simulink model "AFE"  (Simulink 8.7)
settings: Solver=ode23t  StartTime=0  StopTime=.2  MaxStep=.1e-6  RelTol=1e-4  AbsTol=1e-5
InitFcn:
  | clear all
  | VSI_AFE_parameters_G1_s
values from neighbouring files (symbols this model uses):
  Cdc_afe = 105e-6    (= 0.000105)    [VSI_AFE_parameters_G1_s.m]
  DeadTime = 0.5e-6    (= 5e-07)    [VSI_AFE_parameters_G1_s.m]
  f = 400    [VSI_AFE_parameters_G1_s.m]
  Lboost_a = 500e-6    (= 0.0005)    [VSI_AFE_parameters_G1_s.m]
  Lboost_b = 490e-6    (= 0.00049)    [VSI_AFE_parameters_G1_s.m]
  Lboost_c = 510e-6    (= 0.00051)    [VSI_AFE_parameters_G1_s.m]
  LCdc_afe = 0.65e-6    (= 6.5e-07)    [VSI_AFE_parameters_G1_s.m]
  PWM_Cycle = 4000    [VSI_AFE_parameters_G1_s.m]
  RCdc_afe = 0.049    [VSI_AFE_parameters_G1_s.m]
  Rdc = 96    [VSI_AFE_parameters_G1_s.m]
  RLboost_a = 0.080    (= 0.08)    [VSI_AFE_parameters_G1_s.m]
  RLboost_b = 0.084    [VSI_AFE_parameters_G1_s.m]
  RLboost_c = 0.110    (= 0.11)    [VSI_AFE_parameters_G1_s.m]
  Tsw = 1/fsw    (= 5e-05)    [VSI_AFE_parameters_G1_s.m]
  Vfd = 0.75    [VSI_AFE_parameters_G1_s.m]
  Vfs = 1.0    (= 1)    [VSI_AFE_parameters_G1_s.m]
  Vsm = Vse*sqrt(2)    [VSI_AFE_parameters_G1_s.m]
undefined symbols (not defined in the file or in its folder): Cdc, Ldc
libraries: powerlib x28, cstblocks x10, simulink x2
settings Model: Creator=marko  LastModifiedBy=mchssbw3
settings SolverCC: MaxConsecutiveMinStep=10  ZeroCrossAlgorithm=Adaptive  AlgebraicLoopSolver=LineSearch
settings DataIOCC: LimitDataPoints=off  SaveFinalState=on  SignalLoggingSaveFormat=ModelDataLogs
settings OptimizationCC: ExpressionDepthLimit=2147483647
settings DebuggingCC: IgnoredZcDiagnostic=none  SolverPrmCheckMsg=warning  FcnCallInpInsideContextMsg=UseLocalSettings  StateNameClashWarn=warning  StrictBusMsg=Warning
settings GRTTargetCC: CombineOutputUpdateFcns=off  GRTInterface=on

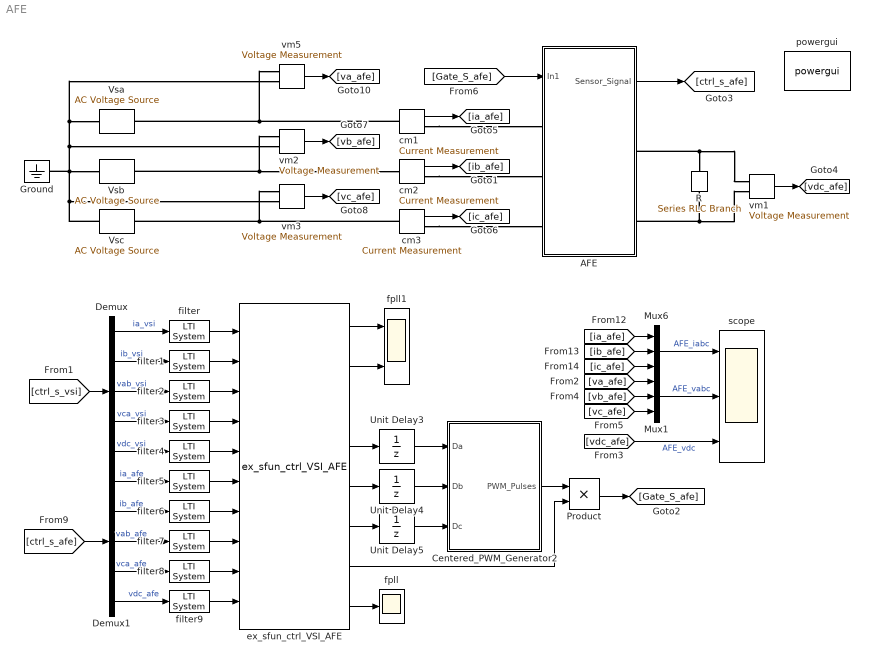
== system AFE ==
  AFE : Subsystem
  Centered_PWM_Generator2 : Subsystem
  Demux : Demux  Outputs=5
  Demux1 : Demux  Outputs=5
  Ground : powerlib/Elements/Ground  LConnTagsString=a
  Mux1 : Mux  Inputs=3
  Mux6 : Mux  Inputs=3
  Product : Product  RndMeth=Zero
  R : powerlib/Elements/Series RLC Branch  LConnTagsString=__new0  RConnTagsString=__new0  BranchType=R  Resistance=Rdc  Inductance=Ldc  SetiL0=off  InitialCurrent=0  Capacitance=Cdc  Setx0=off  InitialVoltage=0  Measurements=None
  Unit Delay3 : UnitDelay  SampleTime=-1
  Unit Delay4 : UnitDelay  SampleTime=-1
  Unit Delay5 : UnitDelay  SampleTime=Tsw
  Vsa : powerlib/Electrical Sources/AC Voltage Source  Amplitude=Vsm  Phase=0  Frequency=f  SampleTime=0  Measurements=None  BusType=swing  Pref=10e3  Qref=0  Qmin=-inf  Qmax=+inf
  Vsb : powerlib/Electrical Sources/AC Voltage Source  Amplitude=Vsm  Phase=0-120  Frequency=f  SampleTime=0  Measurements=None  BusType=swing  Pref=10e3  Qref=0  Qmin=-inf  Qmax=+inf
  Vsc : powerlib/Electrical Sources/AC Voltage Source  Amplitude=Vsm  Phase=0+120  Frequency=f  SampleTime=0  Measurements=None  BusType=swing  Pref=10e3  Qref=0  Qmin=-inf  Qmax=+inf
  cm1 : powerlib/Measurements/Current Measurement  PhasorSimulation=off  OutputType=Complex  PSBequivalent=0
  cm2 : powerlib/Measurements/Current Measurement  PhasorSimulation=off  OutputType=Complex  PSBequivalent=0
  cm3 : powerlib/Measurements/Current Measurement  PhasorSimulation=off  OutputType=Complex  PSBequivalent=0
  ex_sfun_ctrl_VSI_AFE : S-Function  FunctionName=ex_sfun_ctrl_VSI_AFE  SFunctionDeploymentMode=off  EnableBusSupport=off  mask(Legacy Function){SFunctionSpec=void epwm1_isr(double y1[1], double y2[1], double y3[1], double y4[1], double y5[1], double y6[1], double y7[1], double y8[1], double y9[1], double u1, double u2, double u3, double u4, double u5, double u6, double u7, double u8, double u9, double u10), ShowSpec=off}
      mask prompts: ShowSpec "Display function specification"
      mask help:
      | This block allows you to call the legacy functions specified by the following Legacy Code Tool definition:
      | def.SFunctionName = 'ex_sfun_ctrl_VSI_AFE';
      | def.OutputFcnSpec = 'void epwm1_isr(double y1[1], double y2[1], double y3[1], double y4[1], double y5[1], double y6[1], double y7[1], double y8[1], double y9[1], double u1, double u2, double u3, double u4, double u5, double u6, double u7, double u8, double u9, double u10)';
      | def.HeaderFiles = {'math.h'};
      | def.SourceFiles = {'epwm1_isr.c'};
      | def.SampleTime = 5e-005;
      mask Help: <p>This block was generated automatically by the Legacy Code Tool. For detailed help on this tool, call<a href="matlab:legacy_code('help')"> legacy_code('help')</a>.</p>
      mask Callback ShowSpec:
      | if strcmp(get_param(gcbh, 'ShowSpec'), 'on')
      |   set_param(gcbh, 'MaskDisplay', sprintf('fprintf(''%s'');', get_param(gcbh, 'SFunctionSpec')));
      | else
      |   set_param(gcbh, 'MaskDisplay', sprintf('fprintf(''%s'');', get_param(gcbh, 'FunctionName')));
      | end
      mask Display: fprintf('ex_sfun_ctrl_VSI_AFE');
  filter{,1..9} (10 alike) : cstblocks/LTI System  sys=tf_filter  IC=[]
  fpll : Scope
  fpll1 : Scope  NumInputPorts=2
  powergui : powerlib/powergui  Priority=1  SimulationMode=Continuous  SolverType=Tustin  SampleTime=100e-9  frequency=60  SPID=on  DisableSnubberDevices=off  DisableRonSwitches=off  DisableVfSwitches=off  SwTol=0  DisplayEquations=off  Interpol=off  ExternalGateDelay=off  methode=off  Ts=0  FunctionMessages=off  echomessages=off  HookPort=off  EnableUseOfTLC=off  x0status=blocks  frequencyindice=0  Pbase=100e6  ErrMax=1e-4  Iterations=50  UnitsV=kV  UnitsW=MW  buscounter=0  RestoreLinks=warning  ResistiveCurrentMeasurement=off  Frange=[0:2:500]  Ylog=off  Xlog=on  ShowGrid=off  save=off  variable=ZData  structure=iabc  ZoomFFT=off  StartTime=0.1  cycles=2  DisplayStyle=2  fundamental=400  FreqAxis=off  MaxFrequency=100000  frequencyindicesteady=400  RmsSteady=1  display=off
  scope : Scope  NumInputPorts=3
  vm{1..3,5} (4 alike) : powerlib/Measurements/Voltage Measurement  PhasorSimulation=off  OutputType=Complex  PSBequivalent=0
  wires:
  vm5/1 -> [va_afe]
  [ia_afe] -> Mux6/1
  [ib_afe] -> Mux6/2
  [ic_afe] -> Mux6/3
  Mux6/1 -> scope/1  "AFE_iabc"
  Demux/1 -> filter/1  "ia_vsi"
  Demux/2 -> filter1/1  "ib_vsi"
  Demux/3 -> filter2/1  "vab_vsi"
  Demux/4 -> filter3/1  "vca_vsi"
  Demux/5 -> filter4/1  "vdc_vsi"
  [ctrl_s_vsi] -> Demux/1
  Demux1/1 -> filter5/1  "ia_afe"
  Demux1/2 -> filter6/1  "ib_afe"
  Demux1/3 -> filter7/1  "vab_afe"
  Demux1/4 -> filter8/1  "vca_afe"
  Demux1/5 -> filter9/1  "vdc_afe"
  [ctrl_s_afe] -> Demux1/1
  [Gate_S_afe] -> AFE/1(In1)
  AFE/1(Sensor_Signal) -> [ctrl_s_afe]
  Unit Delay3/1 -> Centered_PWM_Generator2/1(Da)
  Unit Delay4/1 -> Centered_PWM_Generator2/2(Db)
  Unit Delay5/1 -> Centered_PWM_Generator2/3(Dc)
  ex_sfun_ctrl_VSI_AFE/4 -> Unit Delay3/1
  ex_sfun_ctrl_VSI_AFE/5 -> Unit Delay4/1
  ex_sfun_ctrl_VSI_AFE/6 -> Unit Delay5/1
  filter/1 -> ex_sfun_ctrl_VSI_AFE/1
  filter1/1 -> ex_sfun_ctrl_VSI_AFE/2
  filter2/1 -> ex_sfun_ctrl_VSI_AFE/3
  filter3/1 -> ex_sfun_ctrl_VSI_AFE/4
  filter4/1 -> ex_sfun_ctrl_VSI_AFE/5
  filter5/1 -> ex_sfun_ctrl_VSI_AFE/6
  filter6/1 -> ex_sfun_ctrl_VSI_AFE/7
  filter7/1 -> ex_sfun_ctrl_VSI_AFE/8
  filter8/1 -> ex_sfun_ctrl_VSI_AFE/9
  filter9/1 -> ex_sfun_ctrl_VSI_AFE/10
  Centered_PWM_Generator2/1(PWM_Pulses) -> Product/1
  Product/1 -> [Gate_S_afe]
  ex_sfun_ctrl_VSI_AFE/7 -> Product/2
  ex_sfun_ctrl_VSI_AFE/8 -> fpll/1
  vm1/1 -> [vdc_afe]
  cm1/1 -> [ia_afe]
  Mux1/1 -> scope/2  "AFE_vabc"
  [vdc_afe] -> scope/3  "AFE_vdc"
  cm2/1 -> [ib_afe]
  cm3/1 -> [ic_afe]
  vm2/1 -> [vb_afe]
  vm3/1 -> [vc_afe]
  [va_afe] -> Mux1/1
  [vb_afe] -> Mux1/2
  [vc_afe] -> Mux1/3
  ex_sfun_ctrl_VSI_AFE/1 -> fpll1/1
  ex_sfun_ctrl_VSI_AFE/2 -> fpll1/2
  connections:
  AFE/RConn2 -- R/RConn1 -- vm1/LConn2
  AFE/RConn1 -- R/LConn1 -- vm1/LConn1
  cm1/RConn1 -- AFE/LConn1
  cm2/RConn1 -- AFE/LConn2
  cm3/RConn1 -- AFE/LConn3
  Vsb/LConn1 -- Ground/LConn1 -- Vsc/LConn1 -- vm3/LConn2 -- Vsa/LConn1 -- vm5/LConn2 -- vm2/LConn2
  Vsa/RConn1 -- cm1/LConn1 -- vm5/LConn1
  Vsb/RConn1 -- vm2/LConn1 -- cm2/LConn1
  Vsc/RConn1 -- cm3/LConn1 -- vm3/LConn1

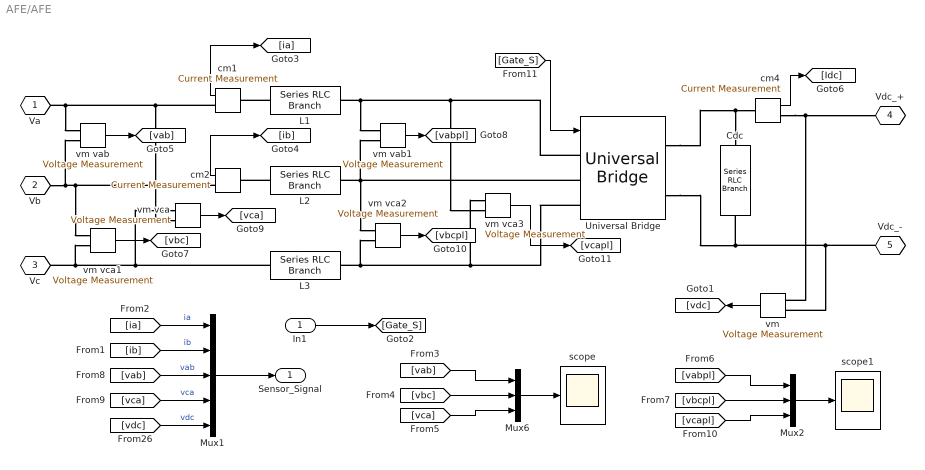
== system AFE/AFE ==
  In1 : Inport
  Cdc : powerlib/Elements/Series RLC Branch  LConnTagsString=__new0  RConnTagsString=__new0  BranchType=RC  Resistance=RCdc_afe  Inductance=LCdc_afe  SetiL0=off  InitialCurrent=0  Capacitance=Cdc_afe  Setx0=off  InitialVoltage=0  Measurements=None
  L1 : powerlib/Elements/Series RLC Branch  LConnTagsString=__new0  RConnTagsString=__new0  BranchType=RL  Resistance=RLboost_a  Inductance=Lboost_a  SetiL0=off  InitialCurrent=0  Capacitance=1e-6  Setx0=off  InitialVoltage=0  Measurements=None
  L2 : powerlib/Elements/Series RLC Branch  LConnTagsString=__new0  RConnTagsString=__new0  BranchType=RL  Resistance=RLboost_b  Inductance=Lboost_b  SetiL0=off  InitialCurrent=0  Capacitance=1e-6  Setx0=off  InitialVoltage=0  Measurements=None
  L3 : powerlib/Elements/Series RLC Branch  LConnTagsString=__new0  RConnTagsString=__new0  BranchType=RL  Resistance=RLboost_c  Inductance=Lboost_c  SetiL0=off  InitialCurrent=0  Capacitance=1e-6  Setx0=off  InitialVoltage=0  Measurements=None
  Mux1 : Mux  Inputs=5
  Mux2 : Mux  Inputs=3
  Mux6 : Mux  Inputs=3
  Universal Bridge : powerlib/Power Electronics/Universal Bridge  Arms=3  SnubberResistance=inf  SnubberCapacitance=inf  Device=IGBT / Diodes  Ron=Rsd  Lon=0  ForwardVoltages=[Vfs Vfd]  ForwardVoltage=0  GTOparameters=[ 10e-6 , 20e-6 ]  IGBTparameters=[ 0, 0 ]  Measurements=None  Measurements_2=None  converterType=Rectifier
  cm1 : powerlib/Measurements/Current Measurement  PhasorSimulation=off  OutputType=Complex  PSBequivalent=0
  cm2 : powerlib/Measurements/Current Measurement  PhasorSimulation=off  OutputType=Complex  PSBequivalent=0
  cm4 : powerlib/Measurements/Current Measurement  PhasorSimulation=off  OutputType=Complex  PSBequivalent=0
  scope : Scope
  scope1 : Scope
  vm : powerlib/Measurements/Voltage Measurement  PhasorSimulation=off  OutputType=Complex  PSBequivalent=0
  vm vab : powerlib/Measurements/Voltage Measurement  PhasorSimulation=off  OutputType=Complex  PSBequivalent=0
  vm vab1 : powerlib/Measurements/Voltage Measurement  PhasorSimulation=off  OutputType=Complex  PSBequivalent=0
  vm vca{,1..3} (4 alike) : powerlib/Measurements/Voltage Measurement  PhasorSimulation=off  OutputType=Complex  PSBequivalent=0
  Va : PMIOPort  Tag=PMCPort  Port=1  Side=Left
  Vb : PMIOPort  Tag=PMCPort  Port=2  Side=Left
  Vc : PMIOPort  Tag=PMCPort  Port=3  Side=Left
  Vdc_+ : PMIOPort  Tag=PMCPort  Port=4  Side=Right
  Vdc_- : PMIOPort  Tag=PMCPort  Port=5  Side=Right
  Sensor_Signal : Outport
  wires:
  [Gate_S] -> Universal Bridge/1
  cm4/1 -> [Idc]
  cm1/1 -> [ia]
  cm2/1 -> [ib]
  vm vab/1 -> [vab]
  vm vca/1 -> [vca]
  vm/1 -> [vdc]
  [ia] -> Mux1/1  "ia"
  [ib] -> Mux1/2  "ib"
  [vab] -> Mux1/3  "vab"
  [vca] -> Mux1/4  "vca"
  [vdc] -> Mux1/5  "vdc"
  Mux1/1 -> Sensor_Signal/1
  In1/1 -> [Gate_S]
  vm vca1/1 -> [vbc]
  vm vab1/1 -> [vabpl]
  vm vca2/1 -> [vbcpl]
  vm vca3/1 -> [vcapl]
  [vab] -> Mux6/1
  [vbc] -> Mux6/2
  [vca] -> Mux6/3
  Mux6/1 -> scope/1
  [vabpl] -> Mux2/1
  [vbcpl] -> Mux2/2
  [vcapl] -> Mux2/3
  Mux2/1 -> scope1/1
  connections:
  Universal Bridge/LConn1 -- L1/RConn1 -- vm vab1/LConn1 -- vm vca3/LConn2
  Universal Bridge/LConn2 -- L2/RConn1 -- vm vca2/LConn1 -- vm vab1/LConn2
  Universal Bridge/LConn3 -- L3/RConn1 -- vm vca2/LConn2 -- vm vca3/LConn1
  vm vab/LConn1 -- cm1/RConn1 -- vm vca/LConn2 -- Va/RConn1
  cm2/RConn1 -- Vb/RConn1 -- vm vab/LConn2 -- vm vca1/LConn1
  cm4/RConn1 -- Vdc_+/RConn1 -- vm/LConn1
  Vdc_-/RConn1 -- Universal Bridge/RConn2 -- Cdc/RConn1 -- vm/LConn2
  L1/LConn1 -- cm1/LConn1
  L2/LConn1 -- cm2/LConn1
  L3/LConn1 -- vm vca/LConn1 -- Vc/RConn1 -- vm vca1/LConn2
  Universal Bridge/RConn1 -- cm4/LConn1 -- Cdc/LConn1

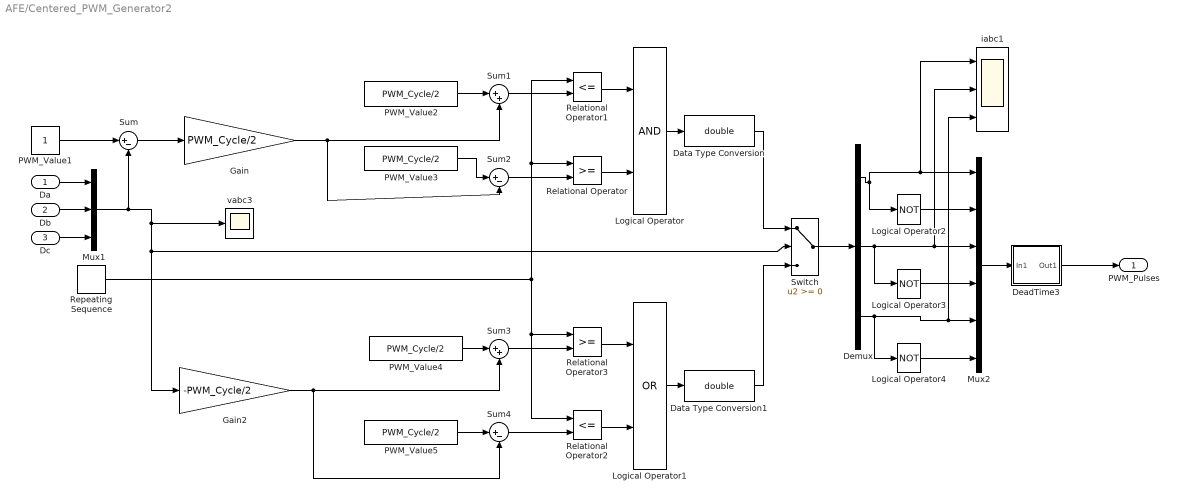
== system AFE/Centered_PWM_Generator2 ==
  Da : Inport
  Db : Inport  Port=2
  Dc : Inport  Port=3
  Data Type Conversion : DataTypeConversion  OutDataTypeStr=double
  Data Type Conversion1 : DataTypeConversion  OutDataTypeStr=double
  DeadTime3 : Subsystem
  Demux : Demux  Outputs=3
  Gain : Gain  Gain=PWM_Cycle/2
  Gain2 : Gain  Gain=-PWM_Cycle/2
  Logical Operator : Logic  AllPortsSameDT=off  OutDataTypeStr=boolean
  Logical Operator1 : Logic  Operator=OR  AllPortsSameDT=off  OutDataTypeStr=boolean
  Logical Operator2 : Logic  Operator=NOT  OutDataTypeStr=float('double')
  Logical Operator3 : Logic  Operator=NOT  OutDataTypeStr=float('double')
  Logical Operator4 : Logic  Operator=NOT  OutDataTypeStr=float('double')
  Mux1 : Mux  Inputs=3
  Mux2 : Mux  Inputs=6
  PWM_Value1 : Constant
  PWM_Value{2..5} (4 alike) : Constant  Value=PWM_Cycle/2
  Relational Operator : RelationalOperator  OutDataTypeStr=boolean
  Relational Operator1 : RelationalOperator  Operator=<=  OutDataTypeStr=boolean
  Relational Operator2 : RelationalOperator  Operator=<=  OutDataTypeStr=boolean
  Relational Operator3 : RelationalOperator  OutDataTypeStr=boolean
  Repeating Sequence : simulink/Sources/Repeating Sequence  rep_seq_t="[0  (PWM_Cycle*12.5e-9)]"  rep_seq_y=[0 PWM_Cycle]
  Sum : Sum  Inputs=|+-
  Sum1 : Sum  Inputs=|++
  Sum2 : Sum  Inputs=|+-
  Sum3 : Sum  Inputs=|++
  Sum4 : Sum  Inputs=|+-
  Switch : Switch
  iabc1 : Scope  NumInputPorts=3
  vabc3 : Scope
  PWM_Pulses : Outport
  wires:
  Logical Operator4/1 -> Mux2/6
  Demux/3 -> Logical Operator4/1, Mux2/5, iabc1/3
  Logical Operator3/1 -> Mux2/4
  Demux/2 -> Logical Operator3/1, Mux2/3, iabc1/2
  Logical Operator2/1 -> Mux2/2
  Demux/1 -> Logical Operator2/1, Mux2/1, iabc1/1
  Mux2/1 -> DeadTime3/1(In1)
  Dc/1 -> Mux1/3
  Db/1 -> Mux1/2
  Da/1 -> Mux1/1
  Mux1/1 -> Sum/2, Switch/2, Gain2/1, vabc3/1
  Switch/1 -> Demux/1
  Data Type Conversion1/1 -> Switch/3
  Gain2/1 -> Sum3/2, Sum4/2
  Logical Operator1/1 -> Data Type Conversion1/1
  Relational Operator2/1 -> Logical Operator1/2
  Relational Operator3/1 -> Logical Operator1/1
  Sum3/1 -> Relational Operator3/2
  Sum4/1 -> Relational Operator2/2
  PWM_Value5/1 -> Sum4/1
  PWM_Value4/1 -> Sum3/1
  Data Type Conversion/1 -> Switch/1
  Logical Operator/1 -> Data Type Conversion/1
  Relational Operator/1 -> Logical Operator/2
  Relational Operator1/1 -> Logical Operator/1
  Sum1/1 -> Relational Operator1/2
  Sum2/1 -> Relational Operator/2
  PWM_Value3/1 -> Sum2/1
  Gain/1 -> Sum2/2, Sum1/2
  Sum/1 -> Gain/1
  PWM_Value1/1 -> Sum/1
  Repeating Sequence/1 -> Relational Operator1/1, Relational Operator/1, Relational Operator3/1, Relational Operator2/1
  DeadTime3/1(Out1) -> PWM_Pulses/1
  PWM_Value2/1 -> Sum1/1

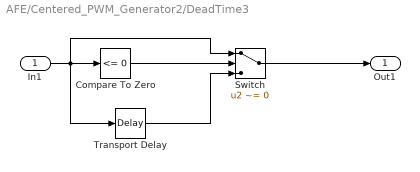
== system AFE/Centered_PWM_Generator2/DeadTime3 ==
  In1 : Inport
  Compare To Zero : simulink/Logic and Bit Operations/Compare To Zero  relop=<=  OutDataTypeStr=uint8
  Switch : Switch  Criteria=u2 ~= 0
  Transport Delay : TransportDelay  DelayTime=DeadTime  BufferSize=2048*16  FixedBuffer=on
  Out1 : Outport
  wires:
  Switch/1 -> Out1/1
  Compare To Zero/1 -> Switch/2
  Transport Delay/1 -> Switch/3
  In1/1 -> Transport Delay/1, Compare To Zero/1, Switch/1
